simulink model "sun_point_SP_power_lib_test"  (R2016b)
settings: Solver=VariableStepAuto  StartTime=0.0  StopTime=5400  RelTol=1e-3
undefined symbols (not defined in the file): fsw_params
libraries: aerolibutil x13, simulink x5, dspmathops x4, vrlib x2, ss_vec_2_angles x2, sun_vector_lib x2, sensor_processing_libs x2, time_conversion_lib x1, MET_lib x1, sgp4_lib_fsw x1, time_coord_rotation_lib x1, mag_vec_LS_lib x1
settings Model: Creator=taylorreynolds  LastModifiedBy=taylorreynolds

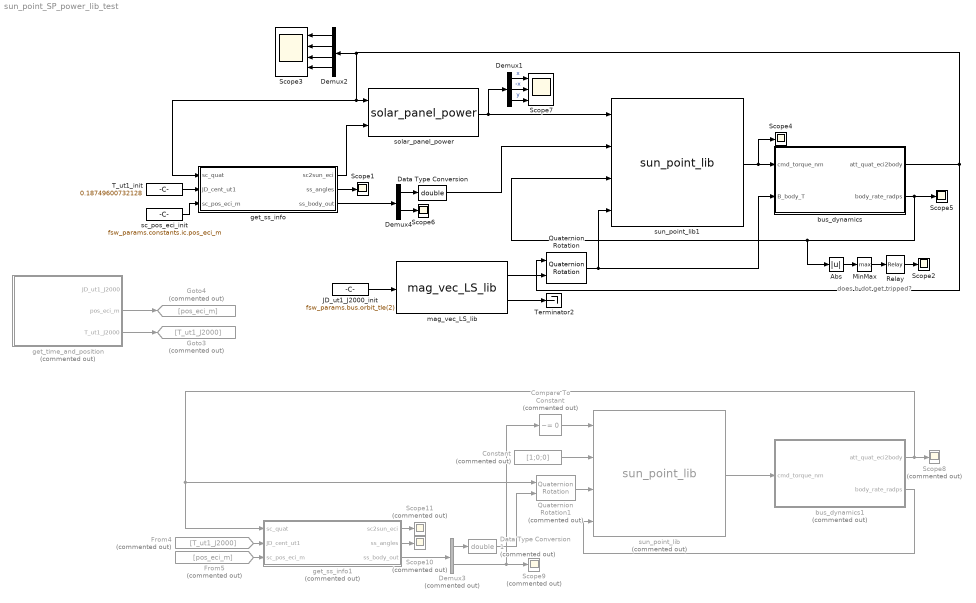
== system sun_point_SP_power_lib_test ==
  note: does b-dot get tripped?
  Abs : Abs
  Compare To Constant : simulink/Logic and Bit Operations/Compare To Constant  Commented=on  relop=~=  const=0  OutDataTypeStr=boolean
  Constant : Constant  Commented=on  Value=[1;0;0]
  Data Type Conversion : DataTypeConversion  OutDataTypeStr=double
  Data Type Conversion1 : DataTypeConversion  Commented=on  OutDataTypeStr=double
  Demux1 : Demux  Outputs=3
  Demux2 : Demux
  Demux3 : Demux  Commented=on  Outputs=[3 1]
  Demux4 : Demux  Outputs=[3 1]
  From4 : From  Commented=on  GotoTag=T_ut1_J2000
  From5 : From  Commented=on  GotoTag=pos_eci_m
  Goto3 : Goto  Commented=on  GotoTag=T_ut1_J2000
  Goto4 : Goto  Commented=on  GotoTag=pos_eci_m
  JD_ut1_J2000_init : Constant  Value=fsw_params.bus.orbit_tle(2)
  MinMax : MinMax  Function=max
  Quaternion Rotation : aerolibutil/Quaternion Rotation
  Quaternion Rotation1 : aerolibutil/Quaternion Rotation  Commented=on
  Relay : Relay  OnSwitchValue=fsw_params.bus.omega_radps_thresh.max  OffSwitchValue=fsw_params.bus.omega_radps_thresh.min
  Scope{1..2,4..6} (5 alike) : Scope
  Scope{8..11} (4 alike) : Scope  Commented=on
  Scope3 : Scope  NumInputPorts=4
  Scope7 : Scope  NumInputPorts=3
  T_ut1_init : Constant  Value=0.18749600732128
  Terminator2 : Terminator
  bus_dynamics : Subsystem
  bus_dynamics1 : Subsystem  Commented=on
  get_ss_info : Subsystem
  get_ss_info1 : Subsystem  Commented=on
  get_time_and_position : Subsystem  Commented=on
  mag_vec_LS_lib : mag_vec_LS_lib/mag_vec_LS_lib
  sc_pos_eci_init : Constant  Value=fsw_params.constants.ic.pos_eci_m
  solar_panel_power : solar_panel_power_lib/solar_panel_power
  sun_point_lib : sun_point_lib/sun_point_lib  Commented=on
  sun_point_lib1 : sun_point_SP_power_lib/sun_point_lib
  wires:
  sun_point_lib1/1 -> Scope4/1, bus_dynamics/1(cmd_torque_nm)
  solar_panel_power/1 -> Demux1/1, sun_point_lib1/1
  Data Type Conversion/1 -> sun_point_lib1/2
  Demux1/2 -> Scope7/2  "-x"
  Demux1/1 -> Scope7/1  "x"
  Demux1/3 -> Scope7/3  "y"
  Demux2/3 -> Scope3/3
  Demux2/4 -> Scope3/4
  Demux2/2 -> Scope3/2
  Demux2/1 -> Scope3/1
  bus_dynamics/1(att_quat_eci2body) -> solar_panel_power/1, get_ss_info/1(sc_quat), Demux2/1, Quaternion Rotation/1
  mag_vec_LS_lib/2 -> Terminator2/1
  Demux4/1 -> Data Type Conversion/1
  Demux4/2 -> Scope6/1
  get_time_and_position/2(pos_eci_m) -> Goto4/1
  get_time_and_position/3(T_ut1_J2000) -> Goto3/1
  T_ut1_init/1 -> get_ss_info/2(JD_cent_ut1)
  get_ss_info/1(sc2sun_eci) -> solar_panel_power/2
  get_ss_info/2(ss_angles) -> Scope1/1
  get_ss_info/3(ss_body_out) -> Demux4/1
  mag_vec_LS_lib/1 -> Quaternion Rotation/2
  Quaternion Rotation/1 -> bus_dynamics/2(B_body_T), sun_point_lib1/4
  bus_dynamics/2(body_rate_radps) -> Scope5/1, Abs/1, sun_point_lib1/3
  Abs/1 -> MinMax/1
  MinMax/1 -> Relay/1
  Relay/1 -> Scope2/1
  sun_point_lib/1 -> bus_dynamics1/1(cmd_torque_nm)
  Constant/1 -> sun_point_lib/2
  Data Type Conversion1/1 -> Quaternion Rotation1/2
  bus_dynamics1/2(body_rate_radps) -> sun_point_lib/4
  bus_dynamics1/1(att_quat_eci2body) -> get_ss_info1/1(sc_quat), Quaternion Rotation1/1, Scope8/1
  Quaternion Rotation1/1 -> sun_point_lib/3
  Compare To Constant/1 -> sun_point_lib/1
  From4/1 -> get_ss_info1/2(JD_cent_ut1)
  From5/1 -> get_ss_info1/3(sc_pos_eci_m)
  get_ss_info1/3(ss_body_out) -> Demux3/1
  Demux3/1 -> Data Type Conversion1/1
  Demux3/2 -> Scope9/1, Compare To Constant/1
  get_ss_info1/2(ss_angles) -> Scope10/1
  get_ss_info1/1(sc2sun_eci) -> Scope11/1
  JD_ut1_J2000_init/1 -> mag_vec_LS_lib/1
  sc_pos_eci_init/1 -> get_ss_info/3(sc_pos_eci_m)

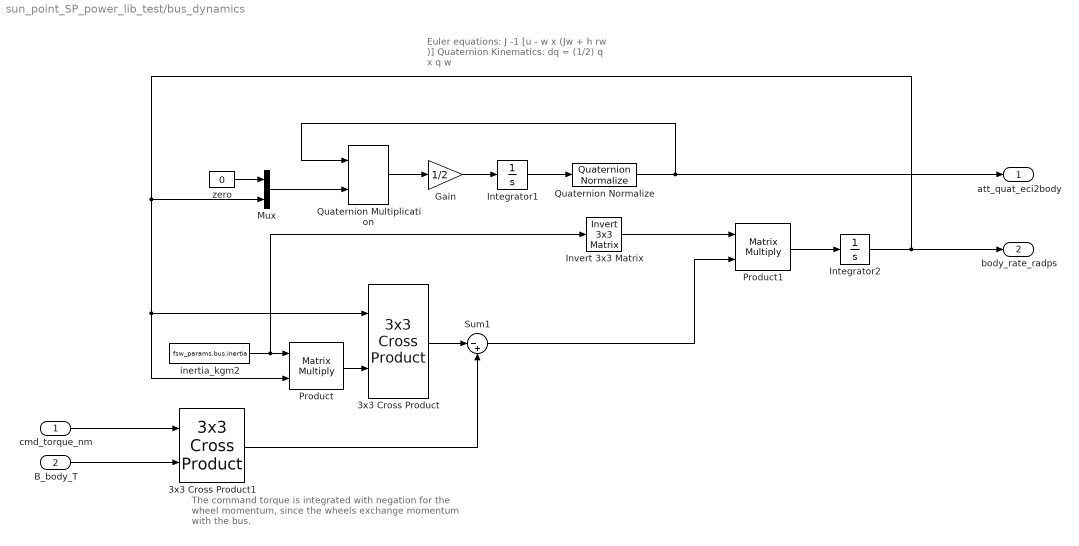
== system sun_point_SP_power_lib_test/bus_dynamics ==
  note: Euler equations: J -1 [u - w x (Jw + h rw )]
      | Quaternion Kinematics: dq = (1/2) q x q w
  note: The command torque is integrated with negation for the wheel
      | momentum, since the wheels exchange momentum with the bus.
  cmd_torque_nm : Inport
  B_body_T : Inport  Port=2
  3x3 Cross Product : aerolibutil/3x3 Cross Product
  3x3 Cross Product1 : aerolibutil/3x3 Cross Product
  Gain : Gain  Gain=1/2
  Integrator1 : Integrator  InitialCondition=sim_params.dynamics.ic.quat_init
      settings: AttributesFormatString=IC: %<InitialCondition>
  Integrator2 : Integrator  InitialCondition=sim_params.dynamics.ic.rate_init
      settings: AttributesFormatString=IC: %<InitialCondition>
  Invert 3x3 Matrix : aerolibutil/Invert  3x3 Matrix
  Mux : Mux  Inputs=[1 3]
  Product : Product  Multiplication=Matrix(*)
  Product1 : Product  Multiplication=Matrix(*)
  Quaternion Multiplication : aerolibutil/Quaternion Multiplication
  Quaternion Normalize : aerolibutil/Quaternion Normalize
  Sum1 : Sum  Inputs=|-+
  inertia_kgm2 : Constant  Value=fsw_params.bus.inertia
  zero : Constant  Value=0
  att_quat_eci2body : Outport
  body_rate_radps : Outport  Port=2
  wires:
  Quaternion Normalize/1 -> att_quat_eci2body/1, Quaternion Multiplication/1
  Integrator2/1 -> body_rate_radps/1, Product/2, 3x3 Cross Product/1, Mux/2
  Product/1 -> 3x3 Cross Product/2
  3x3 Cross Product/1 -> Sum1/1
  Integrator1/1 -> Quaternion Normalize/1
  zero/1 -> Mux/1
  Mux/1 -> Quaternion Multiplication/2
  Quaternion Multiplication/1 -> Gain/1
  Gain/1 -> Integrator1/1
  inertia_kgm2/1 -> Invert 3x3 Matrix/1, Product/1
  Invert 3x3 Matrix/1 -> Product1/1
  Sum1/1 -> Product1/2
  cmd_torque_nm/1 -> 3x3 Cross Product1/1
  Product1/1 -> Integrator2/1
  3x3 Cross Product1/1 -> Sum1/2
  B_body_T/1 -> 3x3 Cross Product1/2

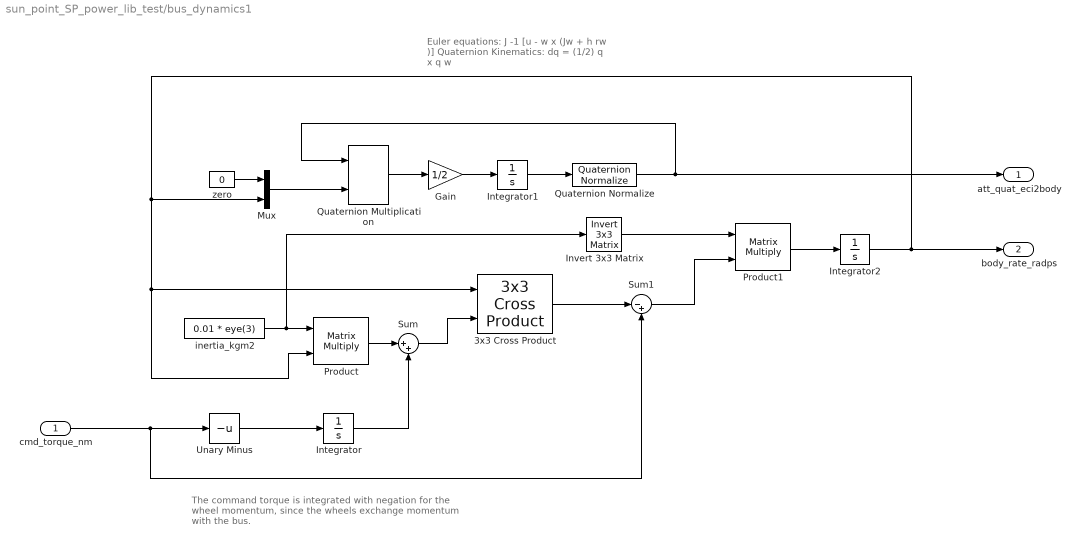
== system sun_point_SP_power_lib_test/bus_dynamics1 ==
  note: Euler equations: J -1 [u - w x (Jw + h rw )]
      | Quaternion Kinematics: dq = (1/2) q x q w
  note: The command torque is integrated with negation for the wheel
      | momentum, since the wheels exchange momentum with the bus.
  cmd_torque_nm : Inport
  3x3 Cross Product : aerolibutil/3x3 Cross Product
  Gain : Gain  Gain=1/2
  Integrator : Integrator  InitialCondition=[0 0 0]
      settings: AttributesFormatString=IC: %<InitialCondition>
  Integrator1 : Integrator  InitialCondition=sim_params.dynamics.ic.quat_init
      settings: AttributesFormatString=IC: %<InitialCondition>
  Integrator2 : Integrator  InitialCondition=[0 0 0]
      settings: AttributesFormatString=IC: %<InitialCondition>
  Invert 3x3 Matrix : aerolibutil/Invert  3x3 Matrix
  Mux : Mux  Inputs=[1 3]
  Product : Product  Multiplication=Matrix(*)
  Product1 : Product  Multiplication=Matrix(*)
  Quaternion Multiplication : aerolibutil/Quaternion Multiplication
  Quaternion Normalize : aerolibutil/Quaternion Normalize
  Sum : Sum  Inputs=|++
  Sum1 : Sum  Inputs=|-+
  Unary Minus : UnaryMinus
  inertia_kgm2 : Constant  Value=0.01 * eye(3)
  zero : Constant  Value=0
  att_quat_eci2body : Outport
  body_rate_radps : Outport  Port=2
  wires:
  Quaternion Normalize/1 -> att_quat_eci2body/1, Quaternion Multiplication/1
  Integrator2/1 -> body_rate_radps/1, 3x3 Cross Product/1, Product/2, Mux/2
  Product/1 -> Sum/1
  Sum/1 -> 3x3 Cross Product/2
  Integrator/1 -> Sum/2
  3x3 Cross Product/1 -> Sum1/1
  Integrator1/1 -> Quaternion Normalize/1
  zero/1 -> Mux/1
  Mux/1 -> Quaternion Multiplication/2
  Quaternion Multiplication/1 -> Gain/1
  Gain/1 -> Integrator1/1
  inertia_kgm2/1 -> Invert 3x3 Matrix/1, Product/1
  Invert 3x3 Matrix/1 -> Product1/1
  Sum1/1 -> Product1/2
  cmd_torque_nm/1 -> Unary Minus/1, Sum1/2
  Product1/1 -> Integrator2/1
  Unary Minus/1 -> Integrator/1

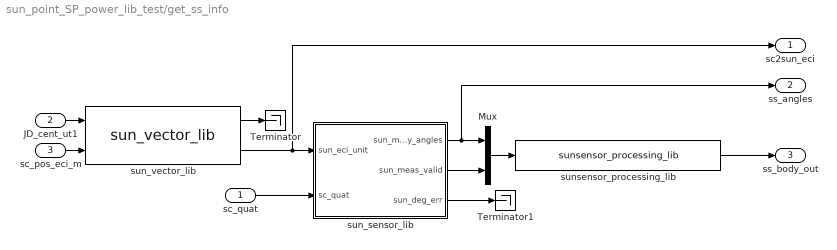
== system sun_point_SP_power_lib_test/get_ss_info ==
  sc_quat : Inport
  JD_cent_ut1 : Inport  Port=2
  sc_pos_eci_m : Inport  Port=3
  Mux : Mux  Inputs=[2 1]
  Terminator : Terminator
  Terminator1 : Terminator
  sun_sensor_lib : Subsystem
  sun_vector_lib : sun_vector_lib/sun_vector_lib
  sunsensor_processing_lib : sensor_processing_libs/sunsensor_processing_lib
  sc2sun_eci : Outport
  ss_angles : Outport  Port=2
  ss_body_out : Outport  Port=3
  wires:
  sun_sensor_lib/2(sun_meas_valid) -> Mux/2
  Mux/1 -> sunsensor_processing_lib/1
  sunsensor_processing_lib/1 -> ss_body_out/1
  sun_vector_lib/2 -> sun_sensor_lib/1(sun_eci_unit), sc2sun_eci/1
  sc_pos_eci_m/1 -> sun_vector_lib/2
  sc_quat/1 -> sun_sensor_lib/2(sc_quat)
  JD_cent_ut1/1 -> sun_vector_lib/1
  sun_sensor_lib/1(sun_meas_body_angles) -> ss_angles/1, Mux/1
  sun_vector_lib/1 -> Terminator/1
  sun_sensor_lib/3(sun_deg_err) -> Terminator1/1

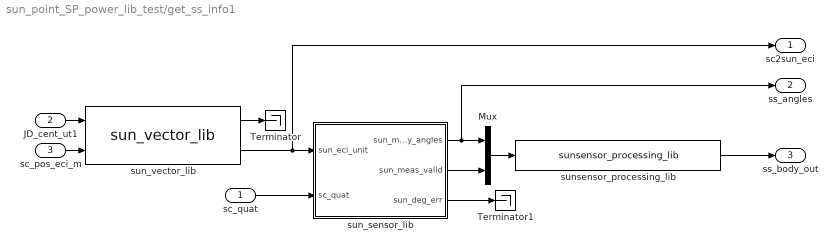
== system sun_point_SP_power_lib_test/get_ss_info1 ==
  sc_quat : Inport
  JD_cent_ut1 : Inport  Port=2
  sc_pos_eci_m : Inport  Port=3
  Mux : Mux  Inputs=[2 1]
  Terminator : Terminator
  Terminator1 : Terminator
  sun_sensor_lib : Subsystem
  sun_vector_lib : sun_vector_lib/sun_vector_lib
  sunsensor_processing_lib : sensor_processing_libs/sunsensor_processing_lib
  sc2sun_eci : Outport
  ss_angles : Outport  Port=2
  ss_body_out : Outport  Port=3
  wires:
  sun_sensor_lib/3(sun_deg_err) -> Terminator1/1
  sun_vector_lib/1 -> Terminator/1
  sun_sensor_lib/1(sun_meas_body_angles) -> Mux/1, ss_angles/1
  JD_cent_ut1/1 -> sun_vector_lib/1
  sc_quat/1 -> sun_sensor_lib/2(sc_quat)
  sc_pos_eci_m/1 -> sun_vector_lib/2
  sun_vector_lib/2 -> sc2sun_eci/1, sun_sensor_lib/1(sun_eci_unit)
  sunsensor_processing_lib/1 -> ss_body_out/1
  Mux/1 -> sunsensor_processing_lib/1
  sun_sensor_lib/2(sun_meas_valid) -> Mux/2

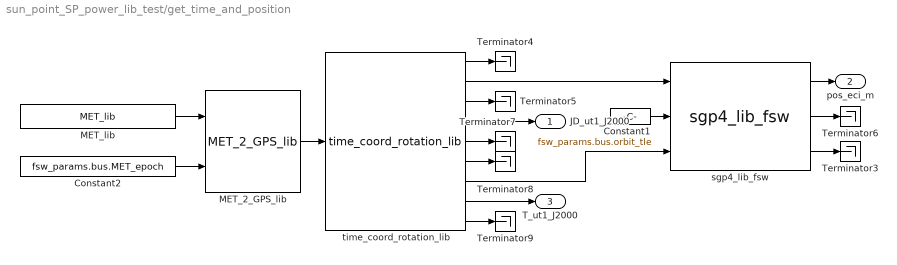
== system sun_point_SP_power_lib_test/get_time_and_position ==
  Constant1 : Constant  Value=fsw_params.bus.orbit_tle
  Constant2 : Constant  Value=fsw_params.bus.MET_epoch
  MET_2_GPS_lib : time_conversion_lib/MET_2_GPS_lib
  MET_lib : MET_lib/MET_lib
  Terminator{3..9} (7 alike) : Terminator
  sgp4_lib_fsw : sgp4_lib_fsw/sgp4_lib_fsw
  time_coord_rotation_lib : time_coord_rotation_lib/time_coord_rotation_lib
  JD_ut1_J2000 : Outport
  pos_eci_m : Outport  Port=2
  T_ut1_J2000 : Outport  Port=3
  wires:
  sgp4_lib_fsw/2 -> Terminator6/1
  time_coord_rotation_lib/6 -> Terminator8/1
  time_coord_rotation_lib/9 -> Terminator9/1
  time_coord_rotation_lib/7 -> sgp4_lib_fsw/3
  Constant2/1 -> MET_2_GPS_lib/2
  MET_2_GPS_lib/1 -> time_coord_rotation_lib/1
  MET_lib/1 -> MET_2_GPS_lib/1
  sgp4_lib_fsw/1 -> pos_eci_m/1
  time_coord_rotation_lib/4 -> JD_ut1_J2000/1
  time_coord_rotation_lib/1 -> Terminator4/1
  time_coord_rotation_lib/3 -> Terminator5/1
  time_coord_rotation_lib/5 -> Terminator7/1
  Constant1/1 -> sgp4_lib_fsw/2
  time_coord_rotation_lib/2 -> sgp4_lib_fsw/1
  sgp4_lib_fsw/3 -> Terminator3/1
  time_coord_rotation_lib/8 -> T_ut1_J2000/1

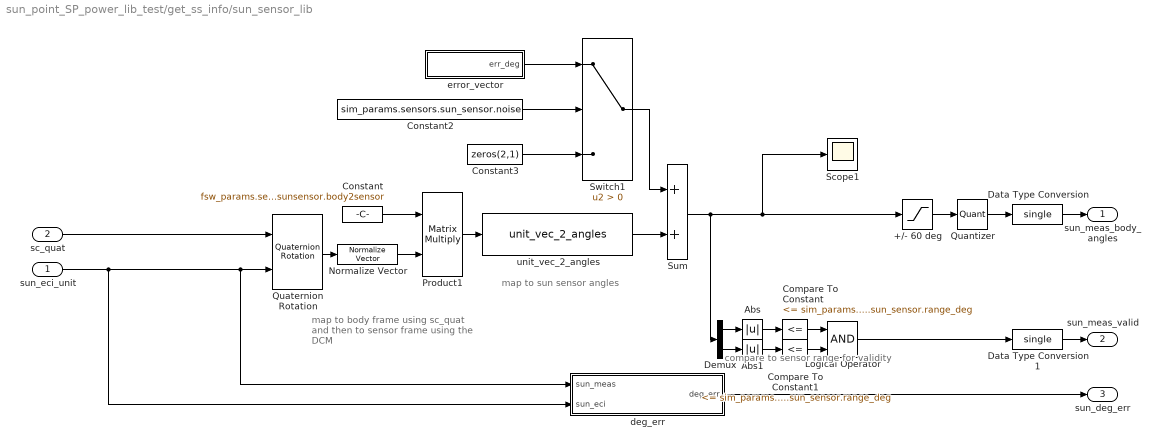
== system sun_point_SP_power_lib_test/get_ss_info/sun_sensor_lib ==
  note: map to sun sensor angles
  note: map to body frame using
      | sc_quat and then to sensor frame
      | using the DCM
  note: compare to sensor range for validity
  sun_eci_unit : Inport
  sc_quat : Inport  Port=2
  +/- 60 deg : Saturate  UpperLimit=60  LowerLimit=-60
  Abs : Abs
  Abs1 : Abs
  Compare To Constant : simulink/Logic and Bit Operations/Compare To Constant  relop=<=  const=sim_params.sensors.sun_sensor.range_deg  OutDataTypeStr=boolean
  Compare To Constant1 : simulink/Logic and Bit Operations/Compare To Constant  relop=<=  const=sim_params.sensors.sun_sensor.range_deg  OutDataTypeStr=boolean
  Constant : Constant  Value=fsw_params.sensor_processing.sunsensor.body2sensor
  Constant2 : Constant  Value=sim_params.sensors.sun_sensor.noise
  Constant3 : Constant  Value=zeros(2,1)
  Data Type Conversion : DataTypeConversion  OutDataTypeStr=single
  Data Type Conversion1 : DataTypeConversion  OutDataTypeStr=single
  Demux : Demux  Outputs=2
  Logical Operator : Logic  AllPortsSameDT=off  OutDataTypeStr=boolean
  Normalize Vector : vrlib/Utilities/Normalize Vector  maxzero=0
  Product1 : Product  Multiplication=Matrix(*)  RndMeth=Zero
  Quantizer : Quantizer  QuantizationInterval=sim_params.sensors.sun_sensor.resolution
  Quaternion Rotation : aerolibutil/Quaternion Rotation
  Scope1 : Scope
  Sum : Sum
  Switch1 : Switch  Criteria=u2 > Threshold
  deg_err : Subsystem
  error_vector : Subsystem
  unit_vec_2_angles : ss_vec_2_angles/unit_vec_2_angles
  sun_meas_body_angles : Outport
  sun_meas_valid : Outport  Port=2
  sun_deg_err : Outport  Port=3
  wires:
  +/- 60 deg/1 -> Quantizer/1
  Data Type Conversion1/1 -> sun_meas_valid/1
  Logical Operator/1 -> Data Type Conversion1/1
  Compare To Constant1/1 -> Logical Operator/2
  Compare To Constant/1 -> Logical Operator/1
  Abs1/1 -> Compare To Constant1/1
  Abs/1 -> Compare To Constant/1
  Demux/2 -> Abs1/1
  Demux/1 -> Abs/1
  Quantizer/1 -> Data Type Conversion/1
  Normalize Vector/1 -> Product1/2
  Data Type Conversion/1 -> sun_meas_body_angles/1
  Quaternion Rotation/1 -> Normalize Vector/1
  error_vector/1("err_deg ") -> Switch1/1
  deg_err/1(deg_err) -> sun_deg_err/1
  sun_eci_unit/1 -> deg_err/1(sun_meas), Quaternion Rotation/2, deg_err/2(sun_eci)
  Switch1/1 -> Sum/1
  Constant3/1 -> Switch1/3
  Constant2/1 -> Switch1/2
  sc_quat/1 -> Quaternion Rotation/1
  Product1/1 -> unit_vec_2_angles/1
  Constant/1 -> Product1/1
  unit_vec_2_angles/1 -> Sum/2
  Sum/1 -> Demux/1, +/- 60 deg/1, Scope1/1

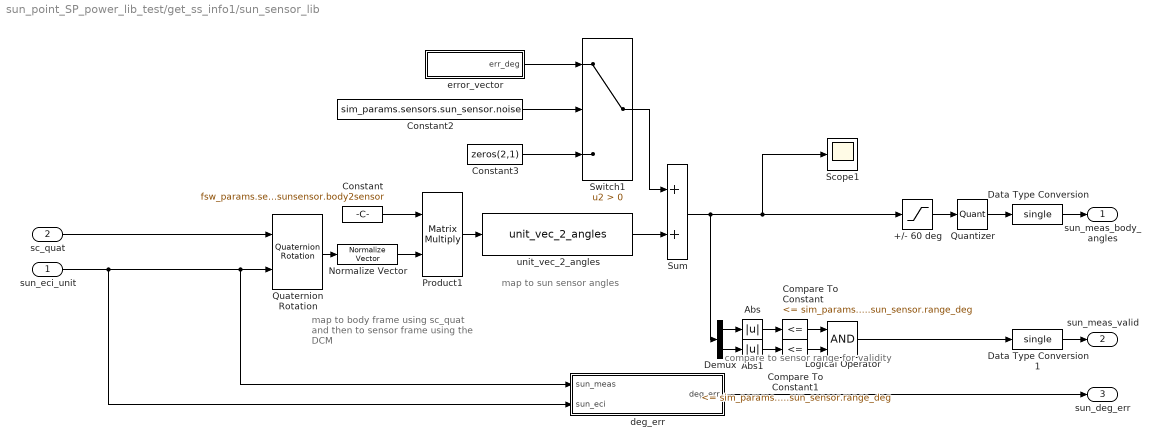
== system sun_point_SP_power_lib_test/get_ss_info1/sun_sensor_lib ==
  note: compare to sensor range for validity
  note: map to body frame using
      | sc_quat and then to sensor frame
      | using the DCM
  note: map to sun sensor angles
  sun_eci_unit : Inport
  sc_quat : Inport  Port=2
  +/- 60 deg : Saturate  UpperLimit=60  LowerLimit=-60
  Abs : Abs
  Abs1 : Abs
  Compare To Constant : simulink/Logic and Bit Operations/Compare To Constant  relop=<=  const=sim_params.sensors.sun_sensor.range_deg  OutDataTypeStr=boolean
  Compare To Constant1 : simulink/Logic and Bit Operations/Compare To Constant  relop=<=  const=sim_params.sensors.sun_sensor.range_deg  OutDataTypeStr=boolean
  Constant : Constant  Value=fsw_params.sensor_processing.sunsensor.body2sensor
  Constant2 : Constant  Value=sim_params.sensors.sun_sensor.noise
  Constant3 : Constant  Value=zeros(2,1)
  Data Type Conversion : DataTypeConversion  OutDataTypeStr=single
  Data Type Conversion1 : DataTypeConversion  OutDataTypeStr=single
  Demux : Demux  Outputs=2
  Logical Operator : Logic  AllPortsSameDT=off  OutDataTypeStr=boolean
  Normalize Vector : vrlib/Utilities/Normalize Vector  maxzero=0
  Product1 : Product  Multiplication=Matrix(*)  RndMeth=Zero
  Quantizer : Quantizer  QuantizationInterval=sim_params.sensors.sun_sensor.resolution
  Quaternion Rotation : aerolibutil/Quaternion Rotation
  Scope1 : Scope
  Sum : Sum
  Switch1 : Switch  Criteria=u2 > Threshold
  deg_err : Subsystem
  error_vector : Subsystem
  unit_vec_2_angles : ss_vec_2_angles/unit_vec_2_angles
  sun_meas_body_angles : Outport
  sun_meas_valid : Outport  Port=2
  sun_deg_err : Outport  Port=3
  wires:
  Sum/1 -> Scope1/1, +/- 60 deg/1, Demux/1
  unit_vec_2_angles/1 -> Sum/2
  Constant/1 -> Product1/1
  Product1/1 -> unit_vec_2_angles/1
  sc_quat/1 -> Quaternion Rotation/1
  Constant2/1 -> Switch1/2
  Constant3/1 -> Switch1/3
  Switch1/1 -> Sum/1
  sun_eci_unit/1 -> deg_err/2(sun_eci), Quaternion Rotation/2, deg_err/1(sun_meas)
  deg_err/1(deg_err) -> sun_deg_err/1
  error_vector/1("err_deg ") -> Switch1/1
  Quaternion Rotation/1 -> Normalize Vector/1
  Data Type Conversion/1 -> sun_meas_body_angles/1
  Normalize Vector/1 -> Product1/2
  Quantizer/1 -> Data Type Conversion/1
  Demux/1 -> Abs/1
  Demux/2 -> Abs1/1
  Abs/1 -> Compare To Constant/1
  Abs1/1 -> Compare To Constant1/1
  Compare To Constant/1 -> Logical Operator/1
  Compare To Constant1/1 -> Logical Operator/2
  Logical Operator/1 -> Data Type Conversion1/1
  Data Type Conversion1/1 -> sun_meas_valid/1
  +/- 60 deg/1 -> Quantizer/1

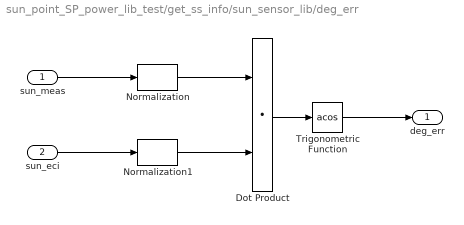
== system sun_point_SP_power_lib_test/get_ss_info/sun_sensor_lib/deg_err ==
  sun_meas : Inport
  sun_eci : Inport  Port=2
  Dot Product : DotProduct  InputSameDT=on  OutDataTypeStr=Inherit: Inherit via internal rule
  Normalization : dspmathops/Normalization  NormType=2-norm  Bias=1e-10  NormOver=Each column  Dimension=1  outputDataTypeStr=Inherit: Same as product output  outputLastDataTypeStr=Inherit: Same as product output  outputMin=[]  outputMax=[]  accumDataTypeStr=Inherit: Same as product output  accumLastDataTypeStr=Inherit: Same as product output  roundingMode=Floor  overflowMode=off
  Normalization1 : dspmathops/Normalization  NormType=2-norm  Bias=1e-10  NormOver=Each column  Dimension=1  outputDataTypeStr=Inherit: Same as product output  outputLastDataTypeStr=Inherit: Same as product output  outputMin=[]  outputMax=[]  accumDataTypeStr=Inherit: Same as product output  accumLastDataTypeStr=Inherit: Same as product output  roundingMode=Floor  overflowMode=off
  Trigonometric Function : Trigonometry  Operator=acos
  deg_err : Outport
  wires:
  Normalization1/1 -> Dot Product/2
  Trigonometric Function/1 -> deg_err/1
  Dot Product/1 -> Trigonometric Function/1
  sun_eci/1 -> Normalization1/1
  Normalization/1 -> Dot Product/1
  sun_meas/1 -> Normalization/1

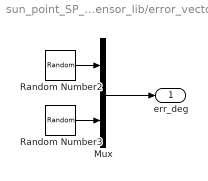
== system sun_point_SP_power_lib_test/get_ss_info/sun_sensor_lib/error_vector ==
  Mux : Mux  Inputs=2
  Random Number2 : RandomNumber  Variance=sim_params.sensors.sun_sensor.deg_err  SampleTime=sim_params.sensors.sun_sensor.sample_time_s
  Random Number3 : RandomNumber  Variance=sim_params.sensors.sun_sensor.deg_err  Seed=1  SampleTime=sim_params.sensors.sun_sensor.sample_time_s
  "err_deg " : Outport
  wires:
  Random Number2/1 -> Mux/1
  Random Number3/1 -> Mux/2
  Mux/1 -> "err_deg "/1

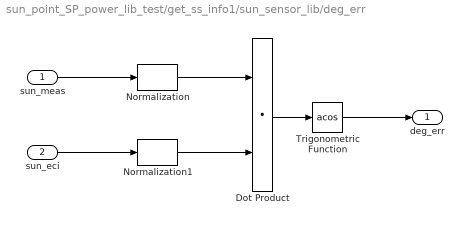
== system sun_point_SP_power_lib_test/get_ss_info1/sun_sensor_lib/deg_err ==
  sun_meas : Inport
  sun_eci : Inport  Port=2
  Dot Product : DotProduct  InputSameDT=on  OutDataTypeStr=Inherit: Inherit via internal rule
  Normalization : dspmathops/Normalization  NormType=2-norm  Bias=1e-10  NormOver=Each column  Dimension=1  outputDataTypeStr=Inherit: Same as product output  outputLastDataTypeStr=Inherit: Same as product output  outputMin=[]  outputMax=[]  accumDataTypeStr=Inherit: Same as product output  accumLastDataTypeStr=Inherit: Same as product output  roundingMode=Floor  overflowMode=off
  Normalization1 : dspmathops/Normalization  NormType=2-norm  Bias=1e-10  NormOver=Each column  Dimension=1  outputDataTypeStr=Inherit: Same as product output  outputLastDataTypeStr=Inherit: Same as product output  outputMin=[]  outputMax=[]  accumDataTypeStr=Inherit: Same as product output  accumLastDataTypeStr=Inherit: Same as product output  roundingMode=Floor  overflowMode=off
  Trigonometric Function : Trigonometry  Operator=acos
  deg_err : Outport
  wires:
  sun_meas/1 -> Normalization/1
  Normalization/1 -> Dot Product/1
  sun_eci/1 -> Normalization1/1
  Dot Product/1 -> Trigonometric Function/1
  Trigonometric Function/1 -> deg_err/1
  Normalization1/1 -> Dot Product/2

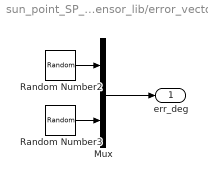
== system sun_point_SP_power_lib_test/get_ss_info1/sun_sensor_lib/error_vector ==
  Mux : Mux  Inputs=2
  Random Number2 : RandomNumber  Variance=sim_params.sensors.sun_sensor.deg_err  SampleTime=sim_params.sensors.sun_sensor.sample_time_s
  Random Number3 : RandomNumber  Variance=sim_params.sensors.sun_sensor.deg_err  Seed=1  SampleTime=sim_params.sensors.sun_sensor.sample_time_s
  "err_deg " : Outport
  wires:
  Mux/1 -> "err_deg "/1
  Random Number3/1 -> Mux/2
  Random Number2/1 -> Mux/1
